simulink model "gm_CustArch_v27"  (R2020a)
settings: Solver=FixedStepDiscrete  StartTime=0.0  StopTime=840000  RelTol=1e-3
libraries: simulink x90, hdlsllib x60, hdlmdlgenlib x2
(part 2 of 2)

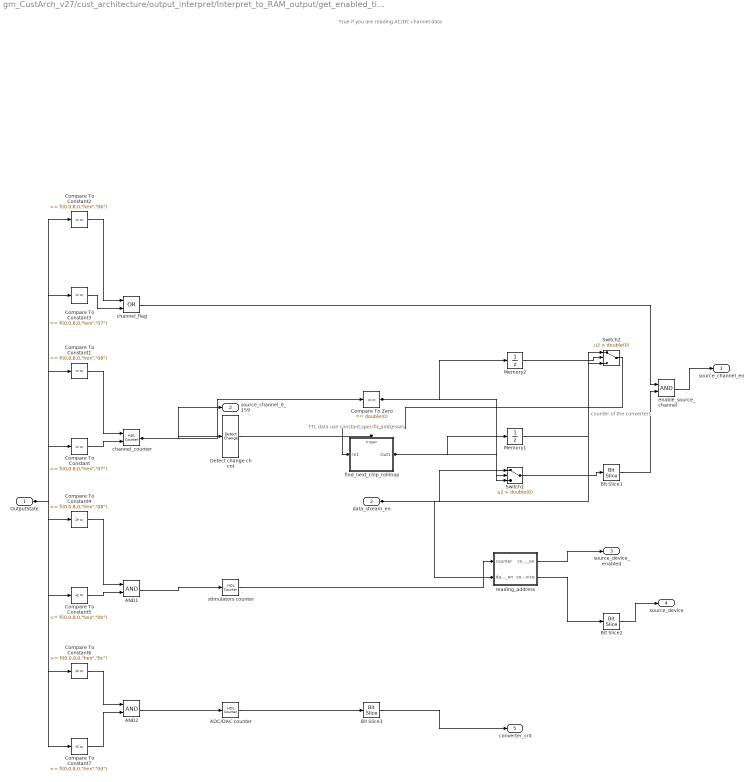
== system gm_CustArch_v27/cust_architecture/output_interpret/Interpret_to_RAM_output/get_enabled_timings  ==
  note: counter of the converters
  note: TTL data use constant specific addresses
  note: True if you are reading AC/DC channel data
  OutputState : Inport  OutDataTypeStr=uint8  PortDimensions=1  SampleTime=1
  data_stream_en : Inport  Port=2  OutDataTypeStr=uint8  PortDimensions=1  SampleTime=1
  ADC/DAC counter : hdlsllib/Sources/HDL Counter  CountType=Count limited  CountInit=double(0)  CountStep=double(1)  CountMax=double(7)  CountFromType=Initial value  CountFrom=double(0)  CountResetPort=off  CountLoadPort=off  CountEnbPort=on  CountDirPort=off  CountDataType=Unsigned  CountWordLen=8  CountFracLen=0  CountSampTime=1
  AND1 : Logic  AllPortsSameDT=off  OutDataTypeStr=boolean  SampleTime=1
  AND2 : Logic  AllPortsSameDT=off  OutDataTypeStr=boolean  SampleTime=1
  Bit Slice1 : hdlsllib/Logic and Bit Operations/Bit Slice  lidx=double(0)  ridx=double(0)
      settings: SourceProductBaseCode=SL
  Bit Slice2 : hdlsllib/Logic and Bit Operations/Bit Slice  lidx=double(2)  ridx=double(0)
      settings: SourceProductBaseCode=SL
  Bit Slice3 : hdlsllib/Logic and Bit Operations/Bit Slice  lidx=double(2)  ridx=double(0)
      settings: SourceProductBaseCode=SL
  Compare To Constant : simulink/Logic and Bit Operations/Compare To Constant  relop===  const="fi(0,0,8,0,\"hex\",\"07\")"  OutDataTypeStr=boolean
  Compare To Constant1 : simulink/Logic and Bit Operations/Compare To Constant  relop===  const="fi(0,0,8,0,\"hex\",\"08\")"  OutDataTypeStr=boolean
  Compare To Constant2 : simulink/Logic and Bit Operations/Compare To Constant  relop===  const="fi(0,0,8,0,\"hex\",\"06\")"  OutDataTypeStr=boolean
  Compare To Constant3 : simulink/Logic and Bit Operations/Compare To Constant  relop===  const="fi(0,0,8,0,\"hex\",\"07\")"  OutDataTypeStr=boolean
  Compare To Constant4 : simulink/Logic and Bit Operations/Compare To Constant  relop=>=  const="fi(0,0,8,0,\"hex\",\"08\")"  OutDataTypeStr=boolean
  Compare To Constant5 : simulink/Logic and Bit Operations/Compare To Constant  relop=<=  const="fi(0,0,8,0,\"hex\",\"0b\")"  OutDataTypeStr=boolean
  Compare To Constant6 : simulink/Logic and Bit Operations/Compare To Constant  relop=>=  const="fi(0,0,8,0,\"hex\",\"0c\")"  OutDataTypeStr=boolean
  Compare To Constant7 : simulink/Logic and Bit Operations/Compare To Constant  relop=<=  const="fi(0,0,8,0,\"hex\",\"0d\")"  OutDataTypeStr=boolean
  Compare To Zero : simulink/Logic and Bit Operations/Compare To Constant  relop===  const=double(0)  OutDataTypeStr=boolean
  Detect change ch cnt : simulink/Logic and Bit Operations/Detect Change  vinit=0  OutDataTypeStr=boolean
  Memory1 : UnitDelay  InitialCondition=double(0)  SampleTime=1
  Memory2 : UnitDelay  InitialCondition=double(0)  SampleTime=1
  Switch1 : Switch  Criteria=u2 > Threshold  Threshold=double(0)  OutDataTypeStr=uint8  SampleTime=1
  Switch2 : Switch  Criteria=u2 > Threshold  Threshold=double(0)  OutDataTypeStr=uint8  SampleTime=1
  channel_counter : hdlsllib/Sources/HDL Counter  CountType=Count limited  CountInit=double(0)  CountStep=double(1)  CountMax=double(159)  CountFromType=Initial value  CountFrom=double(0)  CountResetPort=on  CountLoadPort=off  CountEnbPort=on  CountDirPort=off  CountDataType=Unsigned  CountWordLen=8  CountFracLen=0  CountSampTime=1
  channel_flag : Logic  Operator=OR  AllPortsSameDT=off  OutDataTypeStr=boolean  SampleTime=1
  enable_source_channel : Logic  AllPortsSameDT=off  OutDataTypeStr=boolean  SampleTime=1
  find_next_chip_rollmap : Subsystem
  reading_address : Subsystem
  stimulators counter : hdlsllib/Sources/HDL Counter  CountType=Count limited  CountInit=double(0)  CountStep=double(1)  CountMax=double(7)  CountFromType=Initial value  CountFrom=double(0)  CountResetPort=off  CountLoadPort=off  CountEnbPort=on  CountDirPort=off  CountDataType=Unsigned  CountWordLen=8  CountFracLen=0  CountSampTime=1
  source_channel_en : Outport  VectorParamsAs1DForOutWhenUnconnected=off
  source_channel_0_159 : Outport  Port=2  OutMin=0  OutMax=159  OutDataTypeStr=uint8  VectorParamsAs1DForOutWhenUnconnected=off  LockScale=on
  source_device_enabled : Outport  Port=3  VectorParamsAs1DForOutWhenUnconnected=off
  source_device : Outport  Port=4  VectorParamsAs1DForOutWhenUnconnected=off
  converter_cnt : Outport  Port=5  VectorParamsAs1DForOutWhenUnconnected=off
  wires:
  OutputState/1 -> Compare To Constant7/1, Compare To Constant6/1, Compare To Constant5/1, Compare To Constant4/1, Compare To Constant3/1, Compare To Constant2/1, Compare To Constant1/1, Compare To Constant/1
  data_stream_en/1 -> Switch2/1, Switch1/1, reading_address/2(data_stream_en)
  ADC/DAC counter/1 -> Bit Slice3/1
  AND1/1 -> stimulators counter/1
  AND2/1 -> ADC/DAC counter/1
  Bit Slice1/1 -> enable_source_channel/2
  Bit Slice2/1 -> source_device/1
  Bit Slice3/1 -> converter_cnt/1
  Compare To Constant/1 -> channel_counter/2
  Compare To Constant1/1 -> channel_counter/1
  Compare To Constant2/1 -> channel_flag/1
  Compare To Constant3/1 -> channel_flag/2
  Compare To Constant4/1 -> AND1/1
  Compare To Constant5/1 -> AND1/2
  Compare To Constant6/1 -> AND2/1
  Compare To Constant7/1 -> AND2/2
  Compare To Zero/1 -> Switch1/2, Memory2/1
  Detect change ch cnt/1 -> find_next_chip_rollmap/Trigger
  Memory1/1 -> Switch2/3
  Memory2/1 -> Switch2/2
  Switch1/1 -> Bit Slice1/1
  Switch2/1 -> find_next_chip_rollmap/1(In1)
  channel_counter/1 -> Compare To Zero/1, Detect change ch cnt/1, source_channel_0_159/1
  channel_flag/1 -> enable_source_channel/1
  enable_source_channel/1 -> source_channel_en/1
  find_next_chip_rollmap/1(Out1) -> Switch1/3, Memory1/1
  reading_address/1(source_device_en) -> source_device_enabled/1
  reading_address/2(source_device) -> Bit Slice2/1
  stimulators counter/1 -> reading_address/1("counter ")

== system gm_CustArch_v27/cust_architecture/process_and_retrieve/one_pole_IIR/HP_Butter_1st ==
  Input2 : Inport  OutDataTypeStr=fixdt(1, 16, -3)  PortDimensions=1  SampleTime=1
  Input1 : Inport  Port=2  OutDataTypeStr=fixdt(1, 16, -3)  PortDimensions=1  SampleTime=1
  SumA21 : Sum  Inputs=+-  AccumDataTypeStr=fixdt(1, 17, -3)  OutDataTypeStr=fixdt(1, 16, -3)  RndMeth=Nearest  SaturateOnIntegerOverflow=on  SampleTime=1
  SumB21 : Sum  Inputs=+-  AccumDataTypeStr=fixdt(1, 17, -3)  OutDataTypeStr=fixdt(1, 16, -3)  RndMeth=Nearest  SaturateOnIntegerOverflow=on  SampleTime=1
  a(2)(1) : Gain  Gain="fi(0,1,32,31,\"hex\",\"87ccccc0\")"  ParamDataTypeStr=fixdt(1, 32, 31)  OutDataTypeStr=fixdt(1, 16, -3)  RndMeth=Nearest  SaturateOnIntegerOverflow=on  SampleTime=1
  s(1) : Gain  Gain="fi(0,0,32,32,\"hex\",\"f8333340\")"  ParamDataTypeStr=fixdt(0, 32, 32)  OutDataTypeStr=fixdt(1, 16, -3)  RndMeth=Nearest  SaturateOnIntegerOverflow=on  SampleTime=1
  Output : Outport
  Output1 : Outport  Port=2
  wires:
  Input2/1 -> s(1)/1
  Input1/1 -> SumB21/2, a(2)(1)/1
  SumA21/1 -> SumB21/1, Output1/1
  SumB21/1 -> Output/1
  a(2)(1)/1 -> SumA21/2
  s(1)/1 -> SumA21/1

== system gm_CustArch_v27/cust_architecture/process_and_retrieve/pipe_in_interpret/channel_threshold ==
  th_reading_address : Inport  OutDataTypeStr=fixdt(0, 9, 0)  PortDimensions=1  SampleTime=1
  value_from_pipe_in : Inport  Port=2  OutDataTypeStr=uint16  PortDimensions=1  SampleTime=1
  Bit Slice : hdlsllib/Logic and Bit Operations/Bit Slice  lidx=double(8)  ridx=double(0)
      settings: SourceProductBaseCode=SL
  Compare To Constant : simulink/Logic and Bit Operations/Compare To Constant  relop=<  const="fi(0,0,16,0,\"hex\",\"0140\")"  OutDataTypeStr=boolean
  Delay{,2..5} (5 alike) : Delay  DelayLength=double(1)  InitialCondition=0  SampleTime=1
  Detect Change : simulink/Logic and Bit Operations/Detect Change  vinit=0  OutDataTypeStr=boolean
  Logical Operator : Logic  AllPortsSameDT=off  OutDataTypeStr=boolean  SampleTime=1
  Terminator : Terminator
  th_RAM : hdlsllib/HDL RAMs/Dual Port RAM  ram_size=9
      settings: SourceProductBaseCode=SL
  th : Outport
  wires:
  th_reading_address/1 -> th_RAM/4
  value_from_pipe_in/1 -> Delay5/1, Delay/1, Detect Change/1
  Bit Slice/1 -> Delay4/1
  Compare To Constant/1 -> Delay3/1
  Delay/1 -> Compare To Constant/1, Bit Slice/1
  Delay2/1 -> Logical Operator/1
  Delay3/1 -> Logical Operator/2
  Delay4/1 -> th_RAM/2
  Delay5/1 -> th_RAM/1
  Detect Change/1 -> Delay2/1
  Logical Operator/1 -> th_RAM/3
  th_RAM/1 -> Terminator/1
  th_RAM/2 -> th/1

== system gm_CustArch_v27/cust_architecture/process_and_retrieve/pipe_in_interpret/refractory ==
  value_from_pipe_in : Inport  OutDataTypeStr=uint16  PortDimensions=1  SampleTime=1
  Bit Slice : hdlsllib/Logic and Bit Operations/Bit Slice  lidx=double(1)  ridx=double(0)
      settings: SourceProductBaseCode=SL
  Compare To Constant : simulink/Logic and Bit Operations/Compare To Constant  relop===  const="fi(0,0,16,0,\"hex\",\"0200\")"  OutDataTypeStr=boolean
  Constant : Constant  Value=0  OutDataTypeStr=uint16  SampleTime=1
  Delay{1..4} (4 alike) : Delay  DelayLength=double(1)  InitialCondition=0  SampleTime=1
  Detect Change1 : simulink/Logic and Bit Operations/Detect Change  vinit=0  OutDataTypeStr=boolean
  Logical Operator1 : Logic  AllPortsSameDT=off  OutDataTypeStr=boolean  SampleTime=1
  Terminator : Terminator
  refractory_RAM : hdlsllib/HDL RAMs/Dual Port RAM  ram_size=2
      settings: SourceProductBaseCode=SL
  refractory : Outport
  wires:
  value_from_pipe_in/1 -> Delay4/1, Delay1/1, Detect Change1/1
  Bit Slice/1 -> refractory_RAM/2, refractory_RAM/4
  Compare To Constant/1 -> Delay3/1
  Constant/1 -> Bit Slice/1
  Delay1/1 -> Compare To Constant/1
  Delay2/1 -> Logical Operator1/1
  Delay3/1 -> Logical Operator1/2
  Delay4/1 -> refractory_RAM/1
  Detect Change1/1 -> Delay2/1
  Logical Operator1/1 -> refractory_RAM/3
  refractory_RAM/1 -> Terminator/1
  refractory_RAM/2 -> refractory/1

== system gm_CustArch_v27/cust_architecture/process_and_retrieve/spike_detection/LocalMaxima ==
  filter_output : Inport  OutDataTypeStr=uint16  PortDimensions=1  SampleTime=1
  InputState : Inport  Port=2  OutDataTypeStr=uint8  PortDimensions=1  SampleTime=1
  write porcessing addr = read from storage addr +1 : Inport  Port=3  OutDataTypeStr=fixdt(0, 9, 0)  PortDimensions=1  SampleTime=1
  In4 : Inport  Port=4  OutDataTypeStr=uint16  PortDimensions=1  SampleTime=1
  Compare To Constant : simulink/Logic and Bit Operations/Compare To Constant  relop===  const="fi(0,0,8,0,\"hex\",\"07\")"  OutDataTypeStr=boolean
  Logical Operator1 : Logic  Inputs=3  AllPortsSameDT=off  OutDataTypeStr=boolean  SampleTime=1
  Memory1 : UnitDelay  InitialCondition=double(0)  SampleTime=1
  Memory2 : UnitDelay  InitialCondition=double(0)  SampleTime=1
  Memory4 : UnitDelay  InitialCondition=double(0)  SampleTime=1
  Relational Operator : RelationalOperator  Operator=<=  OutDataTypeStr=boolean  SampleTime=1  RndMeth=Nearest
  Terminator1 : Terminator
  Terminator2 : Terminator
  check_t-1 : RelationalOperator  Operator=<  OutDataTypeStr=boolean  SampleTime=1  RndMeth=Nearest
  check_t-2 : RelationalOperator  Operator=<  OutDataTypeStr=boolean  SampleTime=1  RndMeth=Nearest
  sample_t-1 : hdlsllib/HDL RAMs/Dual Port RAM  ram_size=9
      settings: SourceProductBaseCode=SL
  sample_t-2 : hdlsllib/HDL RAMs/Dual Port RAM  ram_size=9
      settings: SourceProductBaseCode=SL
  local_maxima_out : Outport
  wires:
  filter_output/1 -> check_t-2/2, sample_t-1/1
  InputState/1 -> Compare To Constant/1
  write porcessing addr = read from storage addr +1/1 -> Memory4/1, Memory2/1, sample_t-1/4, sample_t-2/4
  In4/1 -> Relational Operator/2
  Compare To Constant/1 -> Memory1/1
  Logical Operator1/1 -> local_maxima_out/1
  Memory1/1 -> sample_t-1/3, sample_t-2/3
  Memory2/1 -> sample_t-2/2
  Memory4/1 -> sample_t-1/2
  Relational Operator/1 -> Logical Operator1/1
  check_t-1/1 -> Logical Operator1/2
  check_t-2/1 -> Logical Operator1/3
  sample_t-1/1 -> Terminator2/1
  sample_t-1/2 -> check_t-2/1, check_t-1/1, Relational Operator/1, sample_t-2/1
  sample_t-2/1 -> Terminator1/1
  sample_t-2/2 -> check_t-1/2

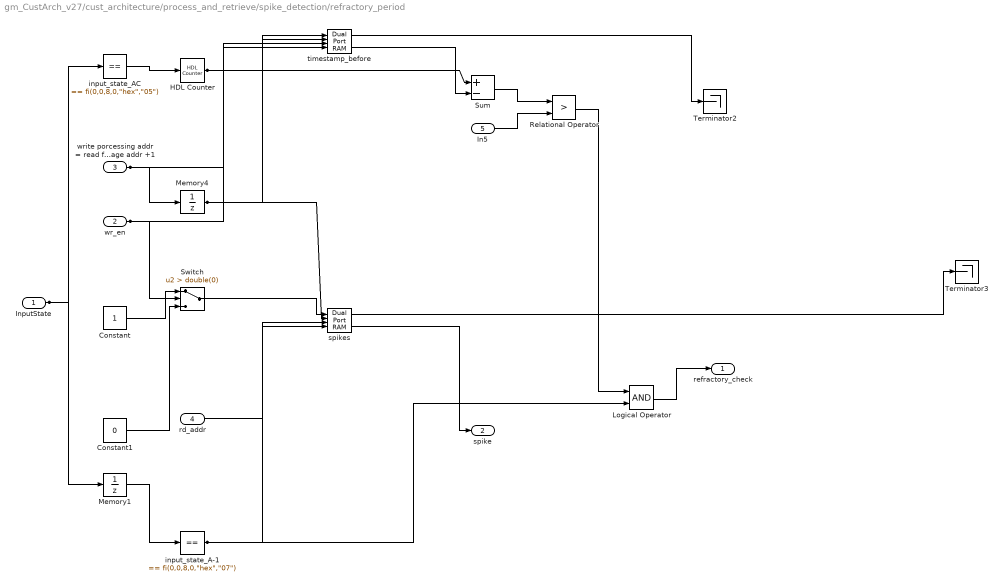
== system gm_CustArch_v27/cust_architecture/process_and_retrieve/spike_detection/refractory_period ==
  InputState : Inport  OutDataTypeStr=uint8  PortDimensions=1  SampleTime=1
  wr_en : Inport  Port=2  OutDataTypeStr=boolean  PortDimensions=1  SampleTime=1
  write porcessing addr = read from storage addr +1 : Inport  Port=3  OutDataTypeStr=fixdt(0, 9, 0)  PortDimensions=1  SampleTime=1
  rd_addr : Inport  Port=4  OutDataTypeStr=fixdt(0, 9, 0)  PortDimensions=1  SampleTime=1
  In5 : Inport  Port=5  OutDataTypeStr=uint16  PortDimensions=1  SampleTime=1
  Constant : Constant  OutDataTypeStr=uint16  SampleTime=1
  Constant1 : Constant  Value=0  OutDataTypeStr=uint16  SampleTime=1
  HDL Counter : hdlsllib/Sources/HDL Counter  CountType=Free running  CountInit=double(0)  CountStep=double(1)  CountMax=25  CountFromType=Initial value  CountFrom=double(0)  CountResetPort=off  CountLoadPort=off  CountEnbPort=on  CountDirPort=off  CountDataType=Unsigned  CountWordLen=32  CountFracLen=0  CountSampTime=1
  Logical Operator : Logic  AllPortsSameDT=off  OutDataTypeStr=boolean  SampleTime=1
  Memory1 : UnitDelay  InitialCondition=double(0)  SampleTime=1
  Memory4 : UnitDelay  InitialCondition=double(0)  SampleTime=1
  Relational Operator : RelationalOperator  Operator=>  OutDataTypeStr=boolean  SampleTime=1  RndMeth=Nearest
  Sum : Sum  Inputs=+-  AccumDataTypeStr=fixdt(1, 33, 0)  OutDataTypeStr=fixdt(1, 33, 0)  SampleTime=1
  Switch : Switch  Criteria=u2 > Threshold  Threshold=double(0)  OutDataTypeStr=uint16  SampleTime=1
  Terminator2 : Terminator
  Terminator3 : Terminator
  input_state_A-1 : simulink/Logic and Bit Operations/Compare To Constant  relop===  const="fi(0,0,8,0,\"hex\",\"07\")"  OutDataTypeStr=boolean
  input_state_AC : simulink/Logic and Bit Operations/Compare To Constant  relop===  const="fi(0,0,8,0,\"hex\",\"05\")"  OutDataTypeStr=boolean
  spikes : hdlsllib/HDL RAMs/Dual Port RAM  ram_size=9
      settings: SourceProductBaseCode=SL
  timestamp_before : hdlsllib/HDL RAMs/Dual Port RAM  ram_size=9
      settings: SourceProductBaseCode=SL
  refractory_check : Outport
  spike : Outport  Port=2
  wires:
  InputState/1 -> input_state_AC/1, Memory1/1
  wr_en/1 -> Switch/2, timestamp_before/3
  write porcessing addr = read from storage addr +1/1 -> Memory4/1, timestamp_before/4
  rd_addr/1 -> spikes/4
  In5/1 -> Relational Operator/2
  Constant/1 -> Switch/1
  Constant1/1 -> Switch/3
  HDL Counter/1 -> Sum/1, timestamp_before/1
  Logical Operator/1 -> refractory_check/1
  Memory1/1 -> input_state_A-1/1
  Memory4/1 -> spikes/2, timestamp_before/2
  Relational Operator/1 -> Logical Operator/1
  Sum/1 -> Relational Operator/1
  Switch/1 -> spikes/1
  input_state_A-1/1 -> Logical Operator/2, spikes/3
  input_state_AC/1 -> HDL Counter/1
  spikes/1 -> Terminator3/1
  spikes/2 -> spike/1
  timestamp_before/1 -> Terminator2/1
  timestamp_before/2 -> Sum/2

== system gm_CustArch_v27/cust_architecture/input_interpret_store_retrieve/Interpret_to_RAM_input/interpret incoming data/condition to count DAC or ADC  ==
  fifo_write_to : Inport  OutDataTypeStr=boolean  PortDimensions=1  SampleTime=1
  input_state : Inport  Port=2  OutDataTypeStr=uint8  PortDimensions=1  SampleTime=1
  AND : Logic  AllPortsSameDT=off  OutDataTypeStr=boolean  SampleTime=1
  OR : Logic  Operator=OR  AllPortsSameDT=off  OutDataTypeStr=boolean  SampleTime=1
  is state_ADC : simulink/Logic and Bit Operations/Compare To Constant  relop===  const="fi(0,0,8,0,\"hex\",\"0d\")"  OutDataTypeStr=boolean
  is state_DAC : simulink/Logic and Bit Operations/Compare To Constant  relop===  const="fi(0,0,8,0,\"hex\",\"0c\")"  OutDataTypeStr=boolean
  Out1 : Outport  VectorParamsAs1DForOutWhenUnconnected=off
  wires:
  fifo_write_to/1 -> AND/1
  input_state/1 -> is state_DAC/1, is state_ADC/1
  AND/1 -> Out1/1
  OR/1 -> AND/2
  is state_ADC/1 -> OR/2
  is state_DAC/1 -> OR/1

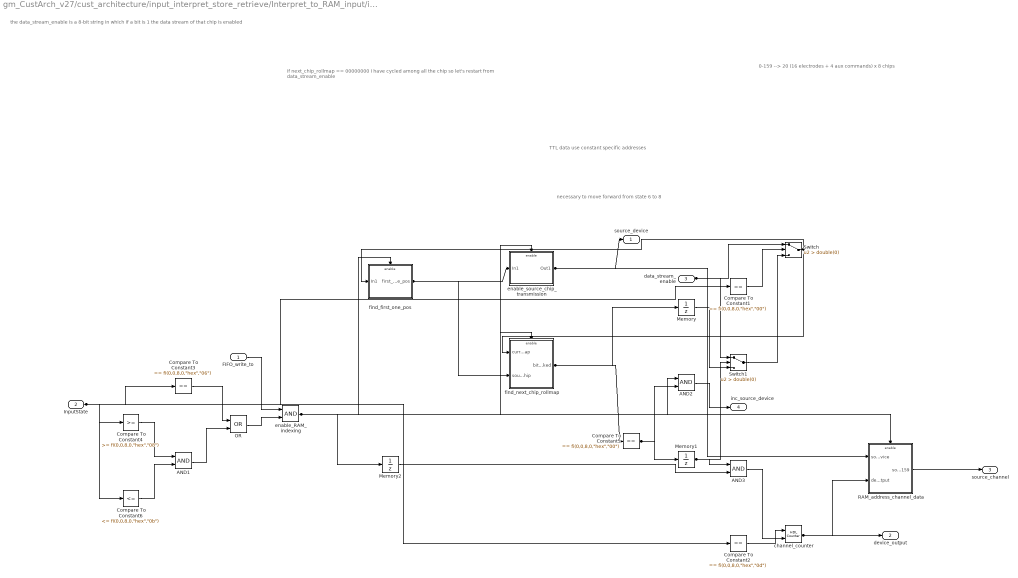
== system gm_CustArch_v27/cust_architecture/input_interpret_store_retrieve/Interpret_to_RAM_input/interpret incoming data/get_sources_and_RAM_addresses ==
  note: TTL data use constant specific addresses
  note: the data_stream_enable is a 8-bit string in which if a bit is 1 the data stream of that chip is enabled
  note: if next_chip_rollmap == 00000000 I have cycled among all the chip so let's restart from data_stream_enable
  note: 0-159 --> 20 (16 electrodes + 4 aux commands) x 8 chips
  note: necessary to move forward from state 6 to 8
  FIFO_write_to : Inport  OutDataTypeStr=boolean  PortDimensions=1  SampleTime=1
  InputState : Inport  Port=2  OutDataTypeStr=uint8  PortDimensions=1  SampleTime=1
  data_stream_enable : Inport  Port=3  OutDataTypeStr=uint8  PortDimensions=1  SampleTime=1
  AND1 : Logic  AllPortsSameDT=off  OutDataTypeStr=boolean  SampleTime=1
  AND2 : Logic  AllPortsSameDT=off  OutDataTypeStr=boolean  SampleTime=1
  AND3 : Logic  AllPortsSameDT=off  OutDataTypeStr=boolean  SampleTime=1
  Compare To Constant1 : simulink/Logic and Bit Operations/Compare To Constant  relop===  const="fi(0,0,8,0,\"hex\",\"00\")"  OutDataTypeStr=boolean
  Compare To Constant2 : simulink/Logic and Bit Operations/Compare To Constant  relop===  const="fi(0,0,8,0,\"hex\",\"0d\")"  OutDataTypeStr=boolean
  Compare To Constant3 : simulink/Logic and Bit Operations/Compare To Constant  relop===  const="fi(0,0,8,0,\"hex\",\"06\")"  OutDataTypeStr=boolean
  Compare To Constant4 : simulink/Logic and Bit Operations/Compare To Constant  relop=>=  const="fi(0,0,8,0,\"hex\",\"08\")"  OutDataTypeStr=boolean
  Compare To Constant5 : simulink/Logic and Bit Operations/Compare To Constant  relop===  const="fi(0,0,8,0,\"hex\",\"00\")"  OutDataTypeStr=boolean
  Compare To Constant6 : simulink/Logic and Bit Operations/Compare To Constant  relop=<=  const="fi(0,0,8,0,\"hex\",\"0b\")"  OutDataTypeStr=boolean
  Memory : UnitDelay  InitialCondition=double(0)  SampleTime=1
  Memory1 : UnitDelay  InitialCondition=double(0)  SampleTime=1
  Memory2 : UnitDelay  InitialCondition=double(0)  SampleTime=1
  OR : Logic  Operator=OR  AllPortsSameDT=off  OutDataTypeStr=boolean  SampleTime=1
  RAM_address_channel_data : Subsystem
  Switch : Switch  Criteria=u2 > Threshold  Threshold=double(0)  OutDataTypeStr=uint8  SampleTime=1
  Switch1 : Switch  Criteria=u2 > Threshold  Threshold=double(0)  OutDataTypeStr=uint8  SampleTime=1
  channel_counter : hdlsllib/Sources/HDL Counter  CountType=Count limited  CountInit=double(0)  CountStep=double(1)  CountMax=double(20)  CountFromType=Initial value  CountFrom=double(0)  CountResetPort=on  CountLoadPort=off  CountEnbPort=on  CountDirPort=off  CountDataType=Unsigned  CountWordLen=8  CountFracLen=0  CountSampTime=1
  enable_RAM_indexing : Logic  AllPortsSameDT=off  OutDataTypeStr=boolean  SampleTime=1
  enable_source_chip_transmission : Subsystem
  find_first_one_pos : Subsystem
  find_next_chip_rollmap : Subsystem
  source_device : Outport  VectorParamsAs1DForOutWhenUnconnected=off
  device_output : Outport  Port=2  VectorParamsAs1DForOutWhenUnconnected=off
  source_channel : Outport  Port=3  VectorParamsAs1DForOutWhenUnconnected=off
  inc_source_device : Outport  Port=4  VectorParamsAs1DForOutWhenUnconnected=off
  wires:
  FIFO_write_to/1 -> enable_RAM_indexing/1
  InputState/1 -> Compare To Constant6/1, Compare To Constant4/1, Compare To Constant3/1, Compare To Constant2/1, Compare To Constant1/1
  data_stream_enable/1 -> Switch1/1, Switch/1
  AND1/1 -> OR/2
  AND2/1 -> inc_source_device/1
  AND3/1 -> channel_counter/2
  Compare To Constant1/1 -> Switch/2
  Compare To Constant2/1 -> channel_counter/1
  Compare To Constant3/1 -> OR/1
  Compare To Constant4/1 -> AND1/1
  Compare To Constant5/1 -> AND2/2, Memory1/1
  Compare To Constant6/1 -> AND1/2
  Memory/1 -> Switch1/3
  Memory1/1 -> Switch1/2, AND3/1
  Memory2/1 -> AND3/2
  OR/1 -> enable_RAM_indexing/2
  RAM_address_channel_data/1(source_channel_0_159) -> source_channel/1
  Switch/1 -> find_next_chip_rollmap/1(curr_chip_rollmap), find_first_one_pos/1(In1)
  Switch1/1 -> Switch/3
  channel_counter/1 -> device_output/1, RAM_address_channel_data/2(dev_output)
  enable_RAM_indexing/1 -> AND2/1, Memory2/1, enable_source_chip_transmission/Enable, RAM_address_channel_data/Enable, find_next_chip_rollmap/Enable, find_first_one_pos/Enable
  enable_source_chip_transmission/1(Out1) -> source_device/1, RAM_address_channel_data/1(source_device)
  find_first_one_pos/1(first_one_pos) -> enable_source_chip_transmission/1(In1), find_next_chip_rollmap/2(source_chip)
  find_next_chip_rollmap/1(bit_masked) -> Compare To Constant5/1, Memory/1

== system gm_CustArch_v27/cust_architecture/output_interpret/Interpret_to_RAM_output/get_enabled_timings /find_next_chip_rollmap ==
  In1 : Inport  OutDataTypeStr=uint8  PortDimensions=1
  Trigger : TriggerPort  VariantControl=(inherit)  PortDimensions=1  OutDataTypeStr=boolean
  Bit Rotate : hdlsllib/Logic and Bit Operations/Bit Rotate  mode=Rotate Right  N=double(1)
      settings: SourceProductBaseCode=SL
  Out1 : Outport  InitialOutput=0  VectorParamsAs1DForOutWhenUnconnected=off
  wires:
  In1/1 -> Bit Rotate/1
  Bit Rotate/1 -> Out1/1

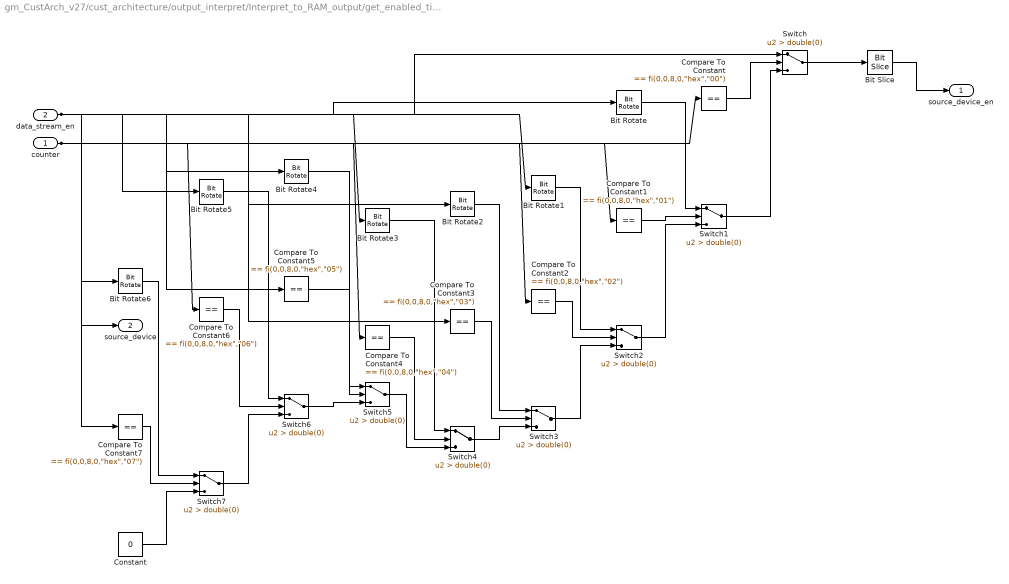
== system gm_CustArch_v27/cust_architecture/output_interpret/Interpret_to_RAM_output/get_enabled_timings /reading_address ==
  "counter " : Inport  OutDataTypeStr=uint8  PortDimensions=1  SampleTime=1
  data_stream_en : Inport  Port=2  OutDataTypeStr=uint8  PortDimensions=1  SampleTime=1
  Bit Rotate : hdlsllib/Logic and Bit Operations/Bit Rotate  mode=Rotate Right  N=double(1)
      settings: SourceProductBaseCode=SL
  Bit Rotate1 : hdlsllib/Logic and Bit Operations/Bit Rotate  mode=Rotate Right  N=double(2)
      settings: SourceProductBaseCode=SL
  Bit Rotate2 : hdlsllib/Logic and Bit Operations/Bit Rotate  mode=Rotate Right  N=double(3)
      settings: SourceProductBaseCode=SL
  Bit Rotate3 : hdlsllib/Logic and Bit Operations/Bit Rotate  mode=Rotate Right  N=double(4)
      settings: SourceProductBaseCode=SL
  Bit Rotate4 : hdlsllib/Logic and Bit Operations/Bit Rotate  mode=Rotate Right  N=double(5)
      settings: SourceProductBaseCode=SL
  Bit Rotate5 : hdlsllib/Logic and Bit Operations/Bit Rotate  mode=Rotate Right  N=double(6)
      settings: SourceProductBaseCode=SL
  Bit Rotate6 : hdlsllib/Logic and Bit Operations/Bit Rotate  mode=Rotate Right  N=double(7)
      settings: SourceProductBaseCode=SL
  Bit Slice : hdlsllib/Logic and Bit Operations/Bit Slice  lidx=double(0)  ridx=double(0)
      settings: SourceProductBaseCode=SL
  Compare To Constant : simulink/Logic and Bit Operations/Compare To Constant  relop===  const="fi(0,0,8,0,\"hex\",\"00\")"  OutDataTypeStr=boolean
  Compare To Constant1 : simulink/Logic and Bit Operations/Compare To Constant  relop===  const="fi(0,0,8,0,\"hex\",\"01\")"  OutDataTypeStr=boolean
  Compare To Constant2 : simulink/Logic and Bit Operations/Compare To Constant  relop===  const="fi(0,0,8,0,\"hex\",\"02\")"  OutDataTypeStr=boolean
  Compare To Constant3 : simulink/Logic and Bit Operations/Compare To Constant  relop===  const="fi(0,0,8,0,\"hex\",\"03\")"  OutDataTypeStr=boolean
  Compare To Constant4 : simulink/Logic and Bit Operations/Compare To Constant  relop===  const="fi(0,0,8,0,\"hex\",\"04\")"  OutDataTypeStr=boolean
  Compare To Constant5 : simulink/Logic and Bit Operations/Compare To Constant  relop===  const="fi(0,0,8,0,\"hex\",\"05\")"  OutDataTypeStr=boolean
  Compare To Constant6 : simulink/Logic and Bit Operations/Compare To Constant  relop===  const="fi(0,0,8,0,\"hex\",\"06\")"  OutDataTypeStr=boolean
  Compare To Constant7 : simulink/Logic and Bit Operations/Compare To Constant  relop===  const="fi(0,0,8,0,\"hex\",\"07\")"  OutDataTypeStr=boolean
  Constant : Constant  Value=0  OutDataTypeStr=uint8  SampleTime=1
  Switch{,1..7} (8 alike) : Switch  Criteria=u2 > Threshold  Threshold=double(0)  OutDataTypeStr=uint8  SampleTime=1
  source_device_en : Outport  VectorParamsAs1DForOutWhenUnconnected=off
  source_device : Outport  Port=2  VectorParamsAs1DForOutWhenUnconnected=off
  wires:
  "counter "/1 -> Compare To Constant7/1, Compare To Constant6/1, Compare To Constant5/1, Compare To Constant4/1, Compare To Constant3/1, Compare To Constant2/1, Compare To Constant1/1, Compare To Constant/1, source_device/1
  data_stream_en/1 -> Switch/1, Bit Rotate6/1, Bit Rotate5/1, Bit Rotate4/1, Bit Rotate3/1, Bit Rotate2/1, Bit Rotate1/1, Bit Rotate/1
  Bit Rotate/1 -> Switch1/1
  Bit Rotate1/1 -> Switch2/1
  Bit Rotate2/1 -> Switch3/1
  Bit Rotate3/1 -> Switch4/1
  Bit Rotate4/1 -> Switch5/1
  Bit Rotate5/1 -> Switch6/1
  Bit Rotate6/1 -> Switch7/1
  Bit Slice/1 -> source_device_en/1
  Compare To Constant/1 -> Switch/2
  Compare To Constant1/1 -> Switch1/2
  Compare To Constant2/1 -> Switch2/2
  Compare To Constant3/1 -> Switch3/2
  Compare To Constant4/1 -> Switch4/2
  Compare To Constant5/1 -> Switch5/2
  Compare To Constant6/1 -> Switch6/2
  Compare To Constant7/1 -> Switch7/2
  Constant/1 -> Switch7/3
  Switch/1 -> Bit Slice/1
  Switch1/1 -> Switch/3
  Switch2/1 -> Switch1/3
  Switch3/1 -> Switch2/3
  Switch4/1 -> Switch3/3
  Switch5/1 -> Switch4/3
  Switch6/1 -> Switch5/3
  Switch7/1 -> Switch6/3

== system gm_CustArch_v27/cust_architecture/input_interpret_store_retrieve/Interpret_to_RAM_input/interpret incoming data/get_sources_and_RAM_addresses/RAM_address_channel_data ==
  source_device : Inport  OutDataTypeStr=uint8  PortDimensions=1  SampleTime=1
  dev_output : Inport  Port=2  OutDataTypeStr=uint8  PortDimensions=1  SampleTime=1
  Enable : EnablePort  OutDataTypeStr=boolean
  Bit Concat : hdlsllib/Logic and Bit Operations/Bit Concat  numInputs=2
  Bit Slice : hdlsllib/Logic and Bit Operations/Bit Slice  lidx=double(4)  ridx=double(0)
      settings: SourceProductBaseCode=SL
  Bit Slice1 : hdlsllib/Logic and Bit Operations/Bit Slice  lidx=double(2)  ridx=double(0)
      settings: SourceProductBaseCode=SL
  source_channel_0_159 : Outport  InitialOutput=0  VectorParamsAs1DForOutWhenUnconnected=off
  wires:
  source_device/1 -> Bit Slice1/1
  dev_output/1 -> Bit Slice/1
  Bit Concat/1 -> source_channel_0_159/1
  Bit Slice/1 -> Bit Concat/1
  Bit Slice1/1 -> Bit Concat/2

== system gm_CustArch_v27/cust_architecture/input_interpret_store_retrieve/Interpret_to_RAM_input/interpret incoming data/get_sources_and_RAM_addresses/enable_source_chip_transmission ==
  In1 : Inport  OutDataTypeStr=uint8  PortDimensions=1  SampleTime=1
  Enable : EnablePort  OutDataTypeStr=boolean
  Out1 : Outport  InitialOutput=0  VectorParamsAs1DForOutWhenUnconnected=off
  wires:
  In1/1 -> Out1/1

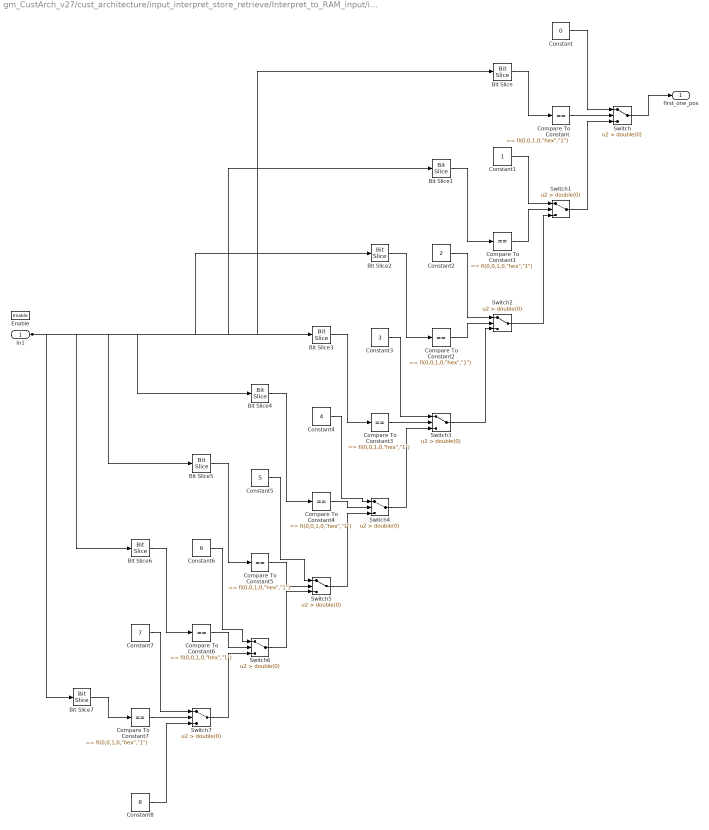
== system gm_CustArch_v27/cust_architecture/input_interpret_store_retrieve/Interpret_to_RAM_input/interpret incoming data/get_sources_and_RAM_addresses/find_first_one_pos ==
  In1 : Inport  OutDataTypeStr=uint8  PortDimensions=1  SampleTime=1
  Enable : EnablePort  OutDataTypeStr=boolean
  Bit Slice : hdlsllib/Logic and Bit Operations/Bit Slice  lidx=double(0)  ridx=double(0)
      settings: SourceProductBaseCode=SL
  Bit Slice1 : hdlsllib/Logic and Bit Operations/Bit Slice  lidx=double(1)  ridx=double(1)
      settings: SourceProductBaseCode=SL
  Bit Slice2 : hdlsllib/Logic and Bit Operations/Bit Slice  lidx=double(2)  ridx=double(2)
      settings: SourceProductBaseCode=SL
  Bit Slice3 : hdlsllib/Logic and Bit Operations/Bit Slice  lidx=double(3)  ridx=double(3)
      settings: SourceProductBaseCode=SL
  Bit Slice4 : hdlsllib/Logic and Bit Operations/Bit Slice  lidx=double(4)  ridx=double(4)
      settings: SourceProductBaseCode=SL
  Bit Slice5 : hdlsllib/Logic and Bit Operations/Bit Slice  lidx=double(5)  ridx=double(5)
      settings: SourceProductBaseCode=SL
  Bit Slice6 : hdlsllib/Logic and Bit Operations/Bit Slice  lidx=double(6)  ridx=double(6)
      settings: SourceProductBaseCode=SL
  Bit Slice7 : hdlsllib/Logic and Bit Operations/Bit Slice  lidx=double(7)  ridx=double(7)
      settings: SourceProductBaseCode=SL
  Compare To Constant{,1..7} (8 alike) : simulink/Logic and Bit Operations/Compare To Constant  relop===  const="fi(0,0,1,0,\"hex\",\"1\")"  OutDataTypeStr=boolean
  Constant : Constant  Value=0  OutDataTypeStr=uint8  SampleTime=1
  Constant1 : Constant  OutDataTypeStr=uint8  SampleTime=1
  Constant2 : Constant  Value=2  OutDataTypeStr=uint8  SampleTime=1
  Constant3 : Constant  Value=3  OutDataTypeStr=uint8  SampleTime=1
  Constant4 : Constant  Value=4  OutDataTypeStr=uint8  SampleTime=1
  Constant5 : Constant  Value=5  OutDataTypeStr=uint8  SampleTime=1
  Constant6 : Constant  Value=6  OutDataTypeStr=uint8  SampleTime=1
  Constant7 : Constant  Value=7  OutDataTypeStr=uint8  SampleTime=1
  Constant8 : Constant  Value=8  OutDataTypeStr=uint8  SampleTime=1
  Switch{,1..7} (8 alike) : Switch  Criteria=u2 > Threshold  Threshold=double(0)  OutDataTypeStr=uint8  SampleTime=1
  first_one_pos : Outport  InitialOutput=0  VectorParamsAs1DForOutWhenUnconnected=off
  wires:
  In1/1 -> Bit Slice7/1, Bit Slice6/1, Bit Slice5/1, Bit Slice4/1, Bit Slice3/1, Bit Slice2/1, Bit Slice1/1, Bit Slice/1
  Bit Slice/1 -> Compare To Constant/1
  Bit Slice1/1 -> Compare To Constant1/1
  Bit Slice2/1 -> Compare To Constant2/1
  Bit Slice3/1 -> Compare To Constant3/1
  Bit Slice4/1 -> Compare To Constant4/1
  Bit Slice5/1 -> Compare To Constant5/1
  Bit Slice6/1 -> Compare To Constant6/1
  Bit Slice7/1 -> Compare To Constant7/1
  Compare To Constant/1 -> Switch/2
  Compare To Constant1/1 -> Switch1/2
  Compare To Constant2/1 -> Switch2/2
  Compare To Constant3/1 -> Switch3/2
  Compare To Constant4/1 -> Switch4/2
  Compare To Constant5/1 -> Switch5/2
  Compare To Constant6/1 -> Switch6/2
  Compare To Constant7/1 -> Switch7/2
  Constant/1 -> Switch/1
  Constant1/1 -> Switch1/1
  Constant2/1 -> Switch2/1
  Constant3/1 -> Switch3/1
  Constant4/1 -> Switch4/1
  Constant5/1 -> Switch5/1
  Constant6/1 -> Switch6/1
  Constant7/1 -> Switch7/1
  Constant8/1 -> Switch7/3
  Switch/1 -> first_one_pos/1
  Switch1/1 -> Switch/3
  Switch2/1 -> Switch1/3
  Switch3/1 -> Switch2/3
  Switch4/1 -> Switch3/3
  Switch5/1 -> Switch4/3
  Switch6/1 -> Switch5/3
  Switch7/1 -> Switch6/3

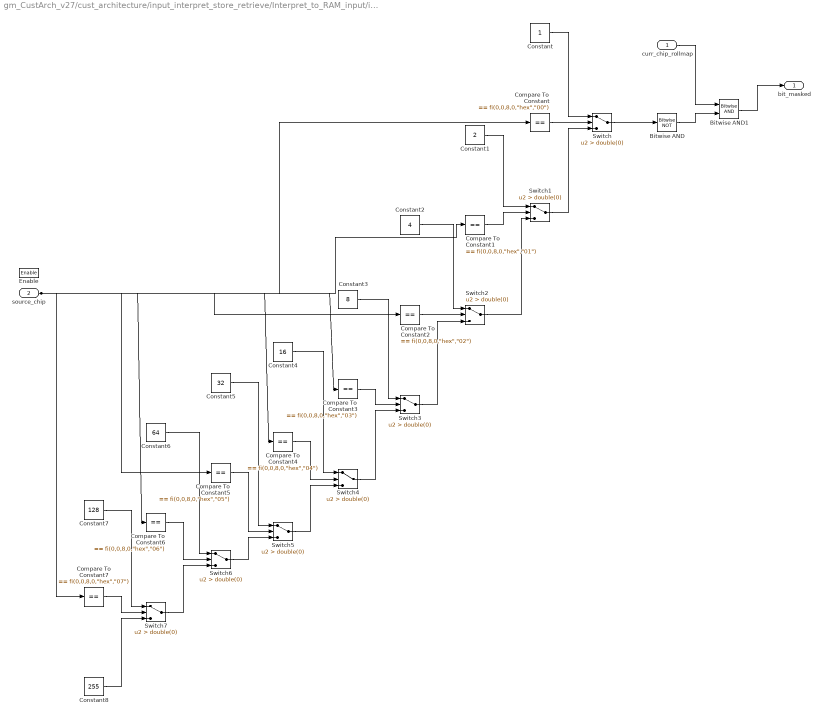
== system gm_CustArch_v27/cust_architecture/input_interpret_store_retrieve/Interpret_to_RAM_input/interpret incoming data/get_sources_and_RAM_addresses/find_next_chip_rollmap ==
  curr_chip_rollmap : Inport  OutDataTypeStr=uint8  PortDimensions=1  SampleTime=1
  source_chip : Inport  Port=2  OutDataTypeStr=uint8  PortDimensions=1  SampleTime=1
  Enable : EnablePort  OutDataTypeStr=boolean
  Bitwise AND : simulink/Logic and Bit Operations/Bitwise Operator  logicop=NOT  UseBitMask=off  BitMask=double(0)  BitMaskRealWorld=Real World Value
  Bitwise AND1 : simulink/Logic and Bit Operations/Bitwise Operator  logicop=AND  UseBitMask=off  NumInputPorts=2  BitMask=double(0)  BitMaskRealWorld=Real World Value
  Compare To Constant : simulink/Logic and Bit Operations/Compare To Constant  relop===  const="fi(0,0,8,0,\"hex\",\"00\")"  OutDataTypeStr=boolean
  Compare To Constant1 : simulink/Logic and Bit Operations/Compare To Constant  relop===  const="fi(0,0,8,0,\"hex\",\"01\")"  OutDataTypeStr=boolean
  Compare To Constant2 : simulink/Logic and Bit Operations/Compare To Constant  relop===  const="fi(0,0,8,0,\"hex\",\"02\")"  OutDataTypeStr=boolean
  Compare To Constant3 : simulink/Logic and Bit Operations/Compare To Constant  relop===  const="fi(0,0,8,0,\"hex\",\"03\")"  OutDataTypeStr=boolean
  Compare To Constant4 : simulink/Logic and Bit Operations/Compare To Constant  relop===  const="fi(0,0,8,0,\"hex\",\"04\")"  OutDataTypeStr=boolean
  Compare To Constant5 : simulink/Logic and Bit Operations/Compare To Constant  relop===  const="fi(0,0,8,0,\"hex\",\"05\")"  OutDataTypeStr=boolean
  Compare To Constant6 : simulink/Logic and Bit Operations/Compare To Constant  relop===  const="fi(0,0,8,0,\"hex\",\"06\")"  OutDataTypeStr=boolean
  Compare To Constant7 : simulink/Logic and Bit Operations/Compare To Constant  relop===  const="fi(0,0,8,0,\"hex\",\"07\")"  OutDataTypeStr=boolean
  Constant : Constant  OutDataTypeStr=uint8  SampleTime=1
  Constant1 : Constant  Value=2  OutDataTypeStr=uint8  SampleTime=1
  Constant2 : Constant  Value=4  OutDataTypeStr=uint8  SampleTime=1
  Constant3 : Constant  Value=8  OutDataTypeStr=uint8  SampleTime=1
  Constant4 : Constant  Value=16  OutDataTypeStr=uint8  SampleTime=1
  Constant5 : Constant  Value=32  OutDataTypeStr=uint8  SampleTime=1
  Constant6 : Constant  Value=64  OutDataTypeStr=uint8  SampleTime=1
  Constant7 : Constant  Value=128  OutDataTypeStr=uint8  SampleTime=1
  Constant8 : Constant  Value=255  OutDataTypeStr=uint8  SampleTime=1
  Switch{,1..7} (8 alike) : Switch  Criteria=u2 > Threshold  Threshold=double(0)  OutDataTypeStr=uint8  SampleTime=1
  bit_masked : Outport  InitialOutput=0  VectorParamsAs1DForOutWhenUnconnected=off
  wires:
  curr_chip_rollmap/1 -> Bitwise AND1/1
  source_chip/1 -> Compare To Constant7/1, Compare To Constant6/1, Compare To Constant5/1, Compare To Constant4/1, Compare To Constant3/1, Compare To Constant2/1, Compare To Constant1/1, Compare To Constant/1
  Bitwise AND/1 -> Bitwise AND1/2
  Bitwise AND1/1 -> bit_masked/1
  Compare To Constant/1 -> Switch/2
  Compare To Constant1/1 -> Switch1/2
  Compare To Constant2/1 -> Switch2/2
  Compare To Constant3/1 -> Switch3/2
  Compare To Constant4/1 -> Switch4/2
  Compare To Constant5/1 -> Switch5/2
  Compare To Constant6/1 -> Switch6/2
  Compare To Constant7/1 -> Switch7/2
  Constant/1 -> Switch/1
  Constant1/1 -> Switch1/1
  Constant2/1 -> Switch2/1
  Constant3/1 -> Switch3/1
  Constant4/1 -> Switch4/1
  Constant5/1 -> Switch5/1
  Constant6/1 -> Switch6/1
  Constant7/1 -> Switch7/1
  Constant8/1 -> Switch7/3
  Switch/1 -> Bitwise AND/1
  Switch1/1 -> Switch/3
  Switch2/1 -> Switch1/3
  Switch3/1 -> Switch2/3
  Switch4/1 -> Switch3/3
  Switch5/1 -> Switch4/3
  Switch6/1 -> Switch5/3
  Switch7/1 -> Switch6/3

== stateflow chart gm_CustArch_v27/cust_architecture/output_interpret/OutputStateMachine/OutputStateMachine ==
  settings: sampleTime=1/1e6  stateMachineType=MOORE_MACHINE  initializeOutput=1
  note: Moore machine
      | State machine to cycle between the different states according
      | to its input variables.
      | The InputState (output of the machine) determines the class of the
      | retrieved data changing its processing in the next steps
  state idle_state
    OutputState=16
  note: The Moore machine output is a function of the current
      | state only. At every time step the input variables dependent
      | on the current state update the output of the state machine.
  state state_magic_number_0
    OutputState=0
  state state_magic_number_01
    OutputState=1
  state state_magic_number_02
    OutputState=2
  state state_magic_number_03
    OutputState=3
  state state_timestamp_0
    OutputState=4
  state state_timestamp_01
    OutputState=5
  state state_DC_sample
    OutputState=6
    count_chs=count_chs+1
  state state_chan_sample
    OutputState=7
  state state_stim_on_off
    OutputState=8
    count_chs=0
    count_stim_on_off=count_stim_on_off+1
  state state_stim_pol
    OutputState=9
    count_stim_on_off=0
    count_stim_pol=count_stim_pol+1
  state state_amp_settle
    OutputState=10
    count_stim_pol=0
    count_amp_settle=count_amp_settle+1
  state state_charge_recov
    OutputState=11
    count_amp_settle=0
    count_state_charge=count_state_charge+1
  state state_DAC
    OutputState=12
    count_state_charge=0
    count_1=count_1+1
  state state_ADC
    OutputState=13
    count_1=0
    count_2=count_2+1
  state state_TTL_in
    count_2=0
    OutputState=14
  state state_TTL_out
    OutputState=15
  (default) -> idle_state
  state_TTL_out -> idle_state
  idle_state -> state_magic_number_0 : [input_state==8]
  state_magic_number_0 -> state_magic_number_01
  state_magic_number_01 -> state_magic_number_02
  state_magic_number_02 -> state_magic_number_03
  state_magic_number_03 -> state_timestamp_0
  state_timestamp_0 -> state_timestamp_01
  state_timestamp_01 -> state_DC_sample
  state_chan_sample -> state_DC_sample [order 1] : [count_chs<160]
  state_DC_sample -> state_chan_sample
  state_chan_sample -> state_stim_on_off [order 2] : [count_chs==160]
  state_stim_on_off -> state_stim_pol : [count_stim_on_off==8]
  state_stim_pol -> state_amp_settle : [count_stim_pol==8]
  state_amp_settle -> state_charge_recov : [count_amp_settle==8]
  state_charge_recov -> state_DAC : [count_state_charge==8]
  state_DAC -> state_DAC [order 2]
  state_DAC -> state_ADC [order 1] : [count_1==8]
  state_ADC -> state_ADC [order 2]
  state_ADC -> state_TTL_in [order 1] : [count_2==8]
  state_TTL_in -> state_TTL_out
  data: OutputState output uint8 =uint8(0); count_1 local uint8 =uint8(0); count_2 local uint8 =uint8(0); input_state input uint8; count_stim_pol local uint8 =uint8(0); count_stim_on_off local uint8 =uint8(0); count_amp_settle local uint8 =uint8(0); count_state_charge local uint8 =uint8(0); count_chs local uint8 =uint8(0)

== stateflow chart gm_CustArch_v27/cust_architecture/input_interpret_store_retrieve/InputStateMachine/InputStateMachine ==
  settings: sampleTime=1/1e6  stateMachineType=MOORE_MACHINE  initializeOutput=1
  note: Moore machine
      | State machine to cycle between the different states according
      | to its input variables.
      | The InputState (output of the machine) determines the class of the
      | retrieved data changing its processing in the next steps
  note: The Moore machine output is a function of the current
      | state only. At every time step the input variables dependent
      | on the current state update the output of the state machine.
  state state_magic_number_0
    InputState=0
  state state_magic_number_01
    InputState=1
  state state_magic_number_02
    InputState=2
  state state_magic_number_03
    InputState=3
  state state_timestamp_0
    InputState=4
  state state_timestamp_01
    InputState=5
  state state_DC_sample
    InputState=6
  state state_chan_sample
    InputState=7
  state state_stim_on_off
    InputState=8
  state state_stim_pol
    InputState=9
  state state_amp_settle
    InputState=10
  state state_charge_recov
    InputState=11
  state state_DAC1
    InputState=12
    count_1=count_1
  state state_DAC
    InputState=12
    count_1=count_1+1
  note: Bad state machine?
      | Probably I should use converter counter but it works
      | so let's keep like this for now
  state state_ADC
    InputState=13
    count_1=0
    count_2=count_2+1
  state state_ADC1
    InputState=13
    count_1=0
    count_2=count_2
  state state_TTL_in
    count_2=0
    InputState=14
  state state_TTL_out
    InputState=15
  (default) -> state_magic_number_0
  state_TTL_out -> state_magic_number_0
  state_magic_number_03 -> state_magic_number_0 [order 2]
  state_timestamp_0 -> state_magic_number_0 [order 2]
  state_magic_number_02 -> state_magic_number_0 [order 2]
  state_magic_number_01 -> state_magic_number_0 [order 2]
  state_magic_number_0 -> state_magic_number_01 : [FIFO_data_in==12043 &  FIFO_write_to==1]
  state_magic_number_01 -> state_magic_number_02 [order 1] : [FIFO_data_in==18801 &  FIFO_write_to==1]
  state_magic_number_02 -> state_magic_number_03 [order 1] : [FIFO_data_in==11402 &  FIFO_write_to==1]
  state_magic_number_03 -> state_timestamp_0 [order 1] : [FIFO_data_in==36180 &  FIFO_write_to==1]
  state_timestamp_0 -> state_timestamp_01 [order 1] : [FIFO_write_to==1]
  state_timestamp_01 -> state_DC_sample : [FIFO_write_to==1]
  state_chan_sample -> state_DC_sample [order 1] : [channel_0_19<20 & FIFO_write_to==1]
  state_DC_sample -> state_stim_on_off [order 2] : [channel_0_19==20 ]
  state_DC_sample -> state_chan_sample [order 1] : [FIFO_write_to==1 & channel_0_19<20]
  state_chan_sample -> state_stim_on_off [order 2] : [channel_0_19==20 & inc_source_device_MSB==1 & FIFO_write_to==1]
  state_stim_on_off -> state_stim_pol : [inc_source_device_MSB==1]
  state_stim_pol -> state_amp_settle : [inc_source_device_MSB==1]
  state_amp_settle -> state_charge_recov : [ inc_source_device_MSB==1]
  state_charge_recov -> state_DAC : [inc_source_device_MSB==1]
  state_DAC -> state_DAC1 [order 3] : [FIFO_write_to==0]
  state_DAC -> state_DAC [order 2] : [FIFO_write_to==1]
  state_DAC1 -> state_DAC : [FIFO_write_to==1]
  state_DAC -> state_ADC [order 1] : [count_1==8]
  state_ADC -> state_ADC1 [order 3] : [FIFO_write_to==0]
  state_ADC -> state_ADC [order 2] : [FIFO_write_to==1]
  state_ADC1 -> state_ADC : [FIFO_write_to==1]
  state_ADC -> state_TTL_in [order 1] : [count_2==8]
  state_TTL_in -> state_TTL_out : [FIFO_write_to==1]
  data: FIFO_data_in input; FIFO_write_to input; InputState output uint8; channel_0_19 input; count_1 local uint8 [0..8] =uint8(0); count_2 local uint8 [0..8] =uint8(0); inc_source_device_MSB input
